simulink model "Halfwave"  (R2023b)
settings: Solver=FixedStepAuto  StartTime=0.0  StopTime=0.1  FixedStep=0.0001  RelTol=1e-3
values from neighbouring files (symbols this model uses):
  capacitance = 0    [matlab.mat]
  frequency = 120    [matlab.mat]
  peakVoltage = 69.0647482014    [matlab.mat]
libraries: spsDiodeLib x5, spsVoltageMeasurementLib x3, spsSeriesRLCBranchLib x2, spsControlledVoltageSourceLib x1, simulink x1, sps_lib x1
settings Model: Creator=Shazin  LastModifiedBy=Shazin

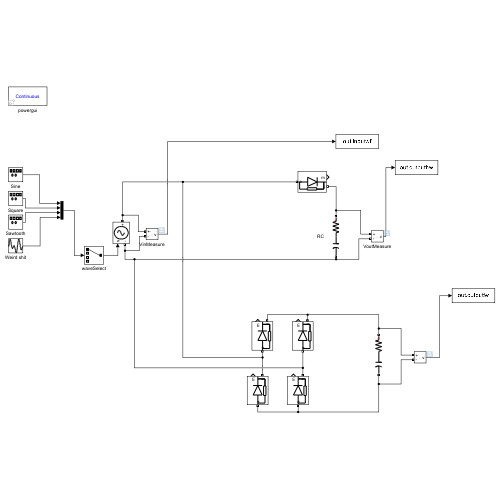
[thumbnail: Simulink's stored preview of the top-level diagram]
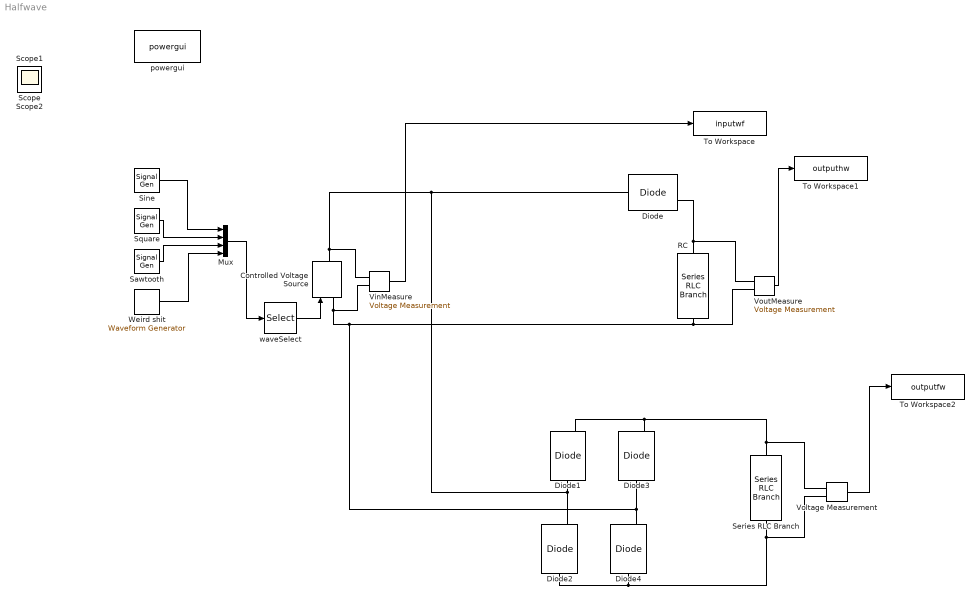
== system Halfwave ==
  Controlled Voltage Source : spsControlledVoltageSourceLib/Controlled Voltage Source  Initialize=on  Source_Type=AC  Amplitude=0  Phase=0  Frequency=0  Measurements=None
  Diode{,1..4} (5 alike) : spsDiodeLib/Diode  Ron=0.001  Lon=0  Vf=0.8  IC=0  UseSnubber=0  Rs=500  Cs=250e-9  Measurements=on
  Mux : Mux
  RC : spsSeriesRLCBranchLib/Series RLC Branch  LConnTagsString=__new0  RConnTagsString=__new0  BranchType=RC  Resistance=1000  Inductance=1e-3  SetiL0=off  InitialCurrent=0  Capacitance=capacitance  Setx0=off  InitialVoltage=0  Measurements=None
  Sawtooth : SignalGenerator  WaveForm=sawtooth  Amplitude=peakVoltage  Frequency=frequency
  Series RLC Branch : spsSeriesRLCBranchLib/Series RLC Branch  LConnTagsString=__new0  RConnTagsString=__new0  BranchType=RC  Resistance=1000  Inductance=1e-3  SetiL0=off  InitialCurrent=0  Capacitance=capacitance  Setx0=off  InitialVoltage=0  Measurements=None
  Sine : SignalGenerator  Amplitude=peakVoltage  Frequency=frequency
  Square : SignalGenerator  WaveForm=square  Amplitude=peakVoltage  Frequency=frequency
  To Workspace : ToWorkspace  VariableName=inputwf  SaveFormat=Timeseries  SampleTime=-1
  To Workspace1 : ToWorkspace  VariableName=outputhw  SaveFormat=Timeseries  SampleTime=-1
  To Workspace2 : ToWorkspace  VariableName=outputfw  SaveFormat=Timeseries  SampleTime=-1
  VinMeasure : spsVoltageMeasurementLib/Voltage Measurement  PhasorSimulation=off  OutputType=Complex  PSBequivalent=0
  Voltage Measurement : spsVoltageMeasurementLib/Voltage Measurement  PhasorSimulation=off  OutputType=Complex  PSBequivalent=0
  VoutMeasure : spsVoltageMeasurementLib/Voltage Measurement  PhasorSimulation=off  OutputType=Complex  PSBequivalent=0
  Weird shit : simulink/Sources/Waveform Generator  OutMin=[]  OutMax=[]  OutDataTypeStr=double  SelectedSignal=1  Signals=sin(peakVoltage*.6, frequency*pi*2*3, 0) + sin(peakVoltage, frequency*pi*2, 0) + sin(peakVoltage, 2*pi*(frequency+20), 50)  BlockNames=MultiportSwitch_ec4f99425d254b4  SampleTime=0.0001
  powergui : sps_lib/powergui  Priority=1  SimulationMode=Continuous  SampleTime=50e-6  frequency=60  Iterations=50  frequencyindice=0  Pbase=100e6  ErrMax=1e-4  UnitsV=kV  UnitsW=MW  buscounter=0  FunctionMessages=off  echomessages=off  EnableUseOfTLC=off  CurrentSourceSwitches=off  DisableSnubberDevices=off  DisableRonSwitches=off  DisableVfSwitches=off  DisplayEquations=off  AutomaticDiscreteSolvers=off  SolverType=Tustin/Backward Euler (TBE)  Interpol=off  ExternalGateDelay=off  methode=off  Ts=100  x0status=blocks  SPID=on  SwTol=0  HookPort=off  NonlinearTolerance=1e-4  nMaxIteration=100  ContinueOnMaxIteration=off  RestoreLinks=warning  ResistiveCurrentMeasurement=off  Frange=[0:2:500]  Ylog=off  Xlog=on  ShowGrid=off  save=off  variable=ZData  structure=0  ZoomFFT=off  StartTime=0.0  cycles=1  DisplayStyle=1  fundamental=60  FreqAxis=off  MaxFrequency=1000  frequencyindicesteady=1  RmsSteady=1  display=off
  waveSelect : Selector  InputPortWidth=4  IndexOptions=Index vector (dialog)  Indices=1  OutputSizes=1
  Scope : Scope
  Scope1 : Scope
  Scope2 : Scope
  wires:
  VoutMeasure/1 -> To Workspace1/1
  VinMeasure/1 -> To Workspace/1
  Sine/1 -> Mux/1
  Square/1 -> Mux/2
  Sawtooth/1 -> Mux/3
  Mux/1 -> waveSelect/1
  waveSelect/1 -> Controlled Voltage Source/1
  Weird shit/1 -> Mux/4
  Voltage Measurement/1 -> To Workspace2/1
  connections:
  Diode/RConn1 -- VoutMeasure/LConn1 -- RC/LConn1
  VinMeasure/LConn1 -- Diode1/LConn1 -- Diode2/RConn1 -- Diode/LConn1 -- Controlled Voltage Source/RConn1
  Controlled Voltage Source/LConn1 -- VinMeasure/LConn2 -- Diode3/LConn1 -- Diode4/RConn1 -- VoutMeasure/LConn2 -- RC/RConn1
  Diode1/RConn1 -- Voltage Measurement/LConn1 -- Series RLC Branch/LConn1 -- Diode3/RConn1
  Diode2/LConn1 -- Voltage Measurement/LConn2 -- Series RLC Branch/RConn1 -- Diode4/LConn1
